simulink model "terrin_Control_Systems"  (R2019a)
settings: Solver=VariableStepAuto  StartTime=0.0  StopTime=400  RelTol=1e-3
libraries: simulink x2
settings Model: Creator=terrin  LastModifiedBy=terrin

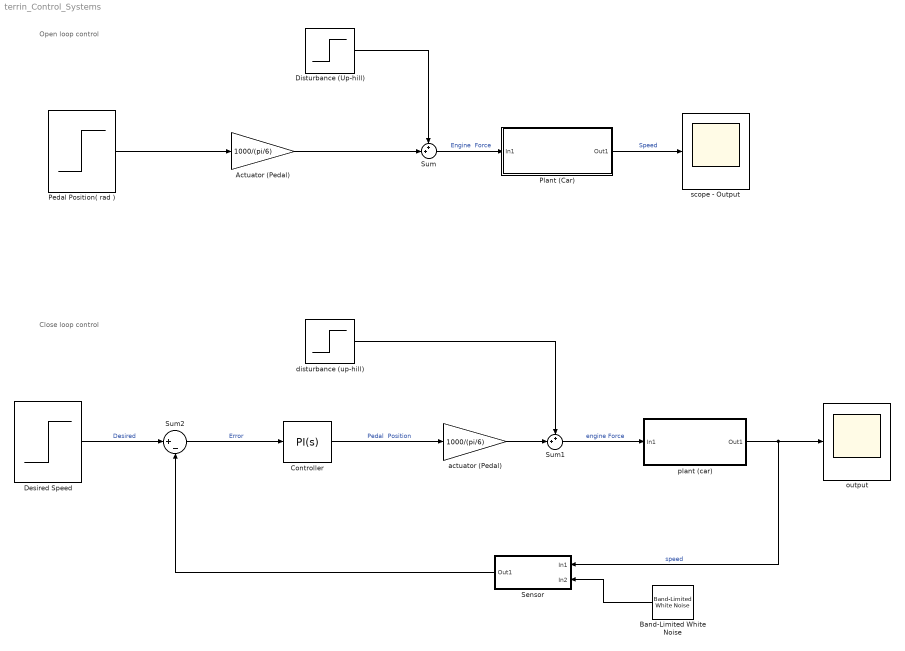
== system terrin_Control_Systems ==
  note: Open loop control
  note: Close loop control
  " Desired Speed" : Step  Time=5  After=20  SampleTime=0
  Actuator (Pedal) : Gain  Gain=1000/(pi/6)
  Band-Limited White Noise : simulink/Sources/Band-Limited White Noise  Cov=[0.01]  Ts=0.1  seed=[23341]
  Controller : simulink/Continuous/PID Controller  Controller=PI  Form=Parallel  TimeDomain=Continuous-time  SampleTime=-1  IntegratorMethod=Forward Euler  FilterMethod=Forward Euler  ControllerParametersSource=internal  P=0.111850088536406  I=0.00559250442682028  D=0  UseFilter=on  N=100  TunerSelectOption=Transfer Function Based (PID Tuner App)  InitialConditionSource=internal  InitialConditionForIntegrator=0  InitialConditionForFilter=0  DifferentiatorICPrevScaledInput=0  ExternalReset=none  TrackingMode=off  Kt=1  LimitOutput=off  UpperSaturationLimit=inf  LowerSaturationLimit=-inf  LinearizeAsGain=on  AntiWindupMode=none  Kb=1  POutMin=[]  POutMax=[]  IOutMin=[]  IOutMax=[]  DOutMin=[]  DOutMax=[]  NOutMin=[]  NOutMax=[]  SumOutMin=[]  SumOutMax=[]  SaturationOutMin=[]  SaturationOutMax=[]  PParamMin=[]  PParamMax=[]  IParamMin=[]  IParamMax=[]  DParamMin=[]  DParamMax=[]  NParamMin=[]  NParamMax=[]  KbParamMin=[]  KbParamMax=[]  KtParamMin=[]  KtParamMax=[]  KbOutMin=[]  KbOutMax=[]  KtOutMin=[]  KtOutMax=[]  IntegratorOutMin=[]  IntegratorOutMax=[]  FilterOutMin=[]  FilterOutMax=[]  SumI1OutMin=[]  SumI1OutMax=[]  SumI2OutMin=[]  SumI2OutMax=[]  SumI3OutMin=[]  SumI3OutMax=[]  SumI4OutMin=[]  SumI4OutMax=[]  SumDOutMin=[]  SumDOutMax=[]  DifferentiatorOutMin=[]  DifferentiatorOutMax=[]  FilterDiffOutCoefMin=[]  FilterDiffOutCoefMax=[]  ReciprocalOutMin=[]  ReciprocalOutMax=[]  SumDenOutMin=[]  SumDenOutMax=[]  SumNumOutMin=[]  SumNumOutMax=[]  DivideOutMin=[]  DivideOutMax=[]  IntegratorContinuousStateAttributes=''  IntegratorStateMustResolveToSignalObject=off  IntegratorRTWStateStorageClass=Auto  FilterContinuousStateAttributes=''  FilterStateMustResolveToSignalObject=off  FilterRTWStateStorageClass=Auto  ParallelPVariant=InternalParameters  IdealPVariant=Disabled  IVariant=InternalParameters  DVariant=Disabled  IntegratorVariant=Continuous  SatVariant=Disabled  AWVariant=Passthrough  PCopyVariant=Disabled  TRVariant=Disabled  FdbkBlocksVariant=Forward  IdealPFdbkVariant=Disabled  SatFdbkVariant=Disabled  DerivativeFilterVariant=Disabled  NVariant=Disabled  NCopyVariant=Disabled_SignalSpec  FilterICVariant=Disabled  IntegratorICVariant=InternalICs  ExternalResetVariant=Disabled  TRSumVariant=Passthrough  SumFdbkVariant=Disabled  SumVariant=Sum_PI
  Disturbance (Up-hill) : Step  Time=200  After=-1000*9.81*sin(pi/45)  SampleTime=0
  Pedal Position( rad ) : Step  Time=5  After=pi/6  SampleTime=0
  Plant (Car) : Subsystem  VariantControlMode=Label  Variant=on  VariantControl=Variant1  LabelModeActiveChoice=Variant1
  Sensor : Subsystem
  Sum : Sum  Inputs=++|
  Sum1 : Sum  Inputs=++|
  Sum2 : Sum  Inputs=|+-
  actuator (Pedal) : Gain  Gain=1000/(pi/6)
  disturbance (up-hill) : Step  Time=200  After=-1000*9.81*sin(pi/45)  SampleTime=0
  output : Scope
  plant (car) : Subsystem  VariantControlMode=Label  Variant=on  VariantControl=Variant1  LabelModeActiveChoice=Variant1
  scope - Output : Scope
  wires:
  Pedal Position( rad )/1 -> Actuator (Pedal)/1
  Actuator (Pedal)/1 -> Sum/2
  plant (car)/1(Out1) -> Sensor/1(In1), output/1  "speed"
  Sum1/1 -> plant (car)/1(In1)  "engine Force"
  actuator (Pedal)/1 -> Sum1/2
  " Desired Speed"/1 -> Sum2/1  "Desired"
  Sensor/1(Out1) -> Sum2/2
  Band-Limited White Noise/1 -> Sensor/2(In2)
  Sum2/1 -> Controller/1  "Error"
  Controller/1 -> actuator (Pedal)/1  "Pedal  Position"
  Sum/1 -> Plant (Car)/1(In1)  "Engine  Force"
  Plant (Car)/1(Out1) -> scope - Output/1  "Speed"
  disturbance (up-hill)/1 -> Sum1/1
  Disturbance (Up-hill)/1 -> Sum/1

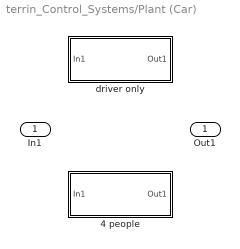
== system terrin_Control_Systems/Plant (Car) ==
  In1 : Inport
  4 people : Subsystem  VariantControl=Choice
  driver only : Subsystem  VariantControl=Variant1
  Out1 : Outport

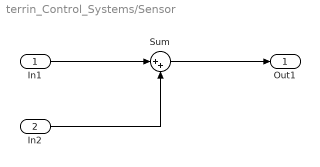
== system terrin_Control_Systems/Sensor ==
  In1 : Inport
  In2 : Inport  Port=2
  Sum : Sum  Inputs=|++
  Out1 : Outport
  wires:
  In1/1 -> Sum/1
  In2/1 -> Sum/2
  Sum/1 -> Out1/1

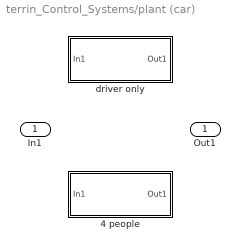
== system terrin_Control_Systems/plant (car) ==
  In1 : Inport
  4 people : Subsystem  VariantControl=Choice
  driver only : Subsystem  VariantControl=Variant1
  Out1 : Outport

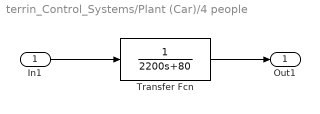
== system terrin_Control_Systems/Plant (Car)/4 people ==
  In1 : Inport
  Transfer Fcn : TransferFcn  Denominator=[2200 80]
  Out1 : Outport
  wires:
  In1/1 -> Transfer Fcn/1
  Transfer Fcn/1 -> Out1/1

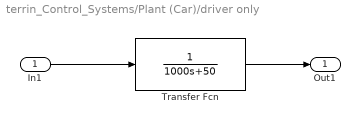
== system terrin_Control_Systems/Plant (Car)/driver only ==
  In1 : Inport
  Transfer Fcn : TransferFcn  Denominator=[1000 50]
  Out1 : Outport
  wires:
  In1/1 -> Transfer Fcn/1
  Transfer Fcn/1 -> Out1/1

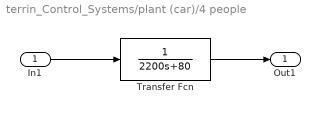
== system terrin_Control_Systems/plant (car)/4 people ==
  In1 : Inport
  Transfer Fcn : TransferFcn  Denominator=[2200 80]
  Out1 : Outport
  wires:
  In1/1 -> Transfer Fcn/1
  Transfer Fcn/1 -> Out1/1

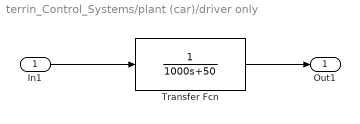
== system terrin_Control_Systems/plant (car)/driver only ==
  In1 : Inport
  Transfer Fcn : TransferFcn  Denominator=[1000 50]
  Out1 : Outport
  wires:
  In1/1 -> Transfer Fcn/1
  Transfer Fcn/1 -> Out1/1
